simulink model "Subsystem"  (R2020b)
settings: Solver=FixedStepAuto  StartTime=0.0  StopTime=3.0  FixedStep=0.06  RelTol=1e-3
settings Model: Creator=nadee  LastModifiedBy=nadee
settings DataIOCC: SaveOutput=off  SaveTime=off

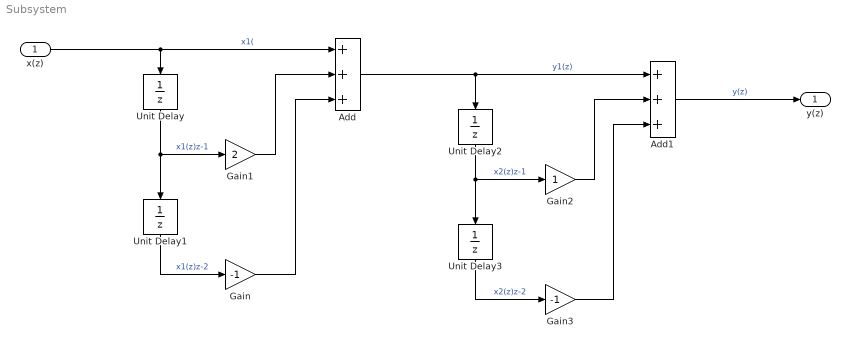
== system Subsystem ==
  x(z) : Inport  OutDataTypeStr=double  PortDimensions=1  SampleTime=[0.059999999999999998,0]
  Add : Sum  Inputs=+++
  Add1 : Sum  Inputs=+++
  Gain : Gain  Gain=-1
  Gain1 : Gain  Gain=2
  Gain2 : Gain
  Gain3 : Gain  Gain=-1
  Unit Delay{,1..3} (4 alike) : UnitDelay  SampleTime=-1  HasFrameUpgradeWarning=on
  y(z) : Outport  OutDataTypeStr=double  PortDimensions=1  SampleTime=[0.059999999999999998,0]
  wires:
  Add/1 -> Add1/1, Unit Delay2/1  "y1(z)"
  Gain/1 -> Add/3
  Gain2/1 -> Add1/2
  Unit Delay/1 -> Unit Delay1/1, Gain1/1  "x1(z)z-1"
  Unit Delay1/1 -> Gain/1  "x1(z)z-2"
  Unit Delay2/1 -> Unit Delay3/1, Gain2/1  "x2(z)z-1"
  Gain1/1 -> Add/2
  x(z)/1 -> Unit Delay/1, Add/1  "x1("
  Unit Delay3/1 -> Gain3/1  "x2(z)z-2"
  Gain3/1 -> Add1/3
  Add1/1 -> y(z)/1  "y(z)"
